simulink model "FSK"  (R2019a)
settings: Solver=VariableStepAuto  StartTime=0.0  StopTime=10.0  MaxStep=0.0001  RelTol=1e-3
libraries: dsparch4 x2, commchan3 x1, commrandsrc3 x1
settings Model: Creator=Lenovo  LastModifiedBy=MOSA

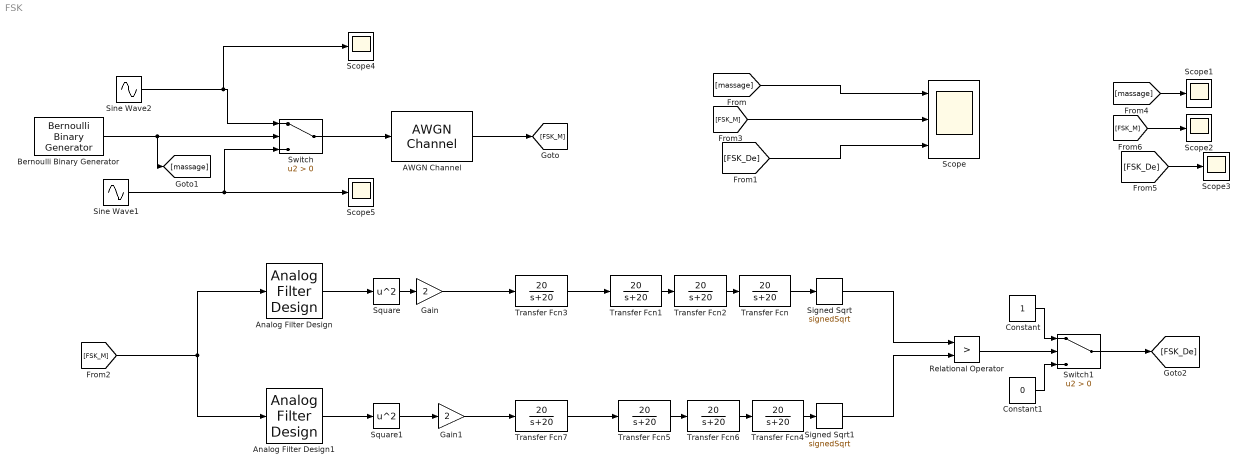
== system FSK ==
  AWGN Channel : commchan3/AWGN Channel  InputProcessing=Columns as channels (frame based)  seed=67  noiseMode="Signal to noise ratio  (SNR)"  EbNodB=10  EsNodB=10  SNRdB=10  bitsPerSym=1  Ps=1  Tsym=1  variance=1
  Analog Filter Design : dsparch4/Analog Filter Design  method=Butterworth  filttype=Bandpass  N=8  Wlo=50  Whi=200  Rp=2  Rs=40
  Analog Filter Design1 : dsparch4/Analog Filter Design  method=Butterworth  filttype=Bandpass  N=8  Wlo=2  Whi=50  Rp=2  Rs=40
  Bernoulli Binary Generator : commrandsrc3/Bernoulli Binary Generator  ProbabilityOfZero=0.5  SeedSource=Parameter  Seed=67  SampleTime=0.4  SamplesPerFrame=1  OutputDataType=double  SimulateUsing=Interpreted execution
  Constant : Constant
  Constant1 : Constant  Value=0
  Gain : Gain  Gain=2
  Gain1 : Gain  Gain=2
  Relational Operator : RelationalOperator  Operator=>  OutDataTypeStr=boolean  RndMeth=Simplest
  Scope : Scope  NumInputPorts=3
  Scope{1..5} (5 alike) : Scope
  Signed Sqrt : Sqrt  Operator=signedSqrt  SaturateOnIntegerOverflow=on
  Signed Sqrt1 : Sqrt  Operator=signedSqrt  SaturateOnIntegerOverflow=on
  Sine Wave1 : Sin  Frequency=31.4  SampleTime=0
  Sine Wave2 : Sin  Frequency=94.2  SampleTime=0
  Square : Math  Operator=square  SaturateOnIntegerOverflow=on
  Square1 : Math  Operator=square  SaturateOnIntegerOverflow=on
  Switch : Switch  Criteria=u2 > Threshold
  Switch1 : Switch  Criteria=u2 > Threshold
  Transfer Fcn{,1..7} (8 alike) : TransferFcn  Numerator=[20]  Denominator=[1 20]
  wires:
  Sine Wave2/1 -> Scope4/1, Switch/1
  Bernoulli Binary Generator/1 -> Switch/2, [massage]
  Sine Wave1/1 -> Switch/3, Scope5/1
  Square/1 -> Gain/1
  Transfer Fcn/1 -> Signed Sqrt/1
  Transfer Fcn1/1 -> Transfer Fcn2/1
  Transfer Fcn2/1 -> Transfer Fcn/1
  Gain/1 -> Transfer Fcn3/1
  Transfer Fcn6/1 -> Transfer Fcn4/1
  Transfer Fcn4/1 -> Signed Sqrt1/1
  Transfer Fcn5/1 -> Transfer Fcn6/1
  Square1/1 -> Gain1/1
  Gain1/1 -> Transfer Fcn7/1
  Analog Filter Design1/1 -> Square1/1
  Analog Filter Design/1 -> Square/1
  Constant/1 -> Switch1/1
  Constant1/1 -> Switch1/3
  Relational Operator/1 -> Switch1/2
  [FSK_M] -> Analog Filter Design/1, Analog Filter Design1/1
  Switch1/1 -> [FSK_De]
  Switch/1 -> AWGN Channel/1
  Transfer Fcn7/1 -> Transfer Fcn5/1
  Transfer Fcn3/1 -> Transfer Fcn1/1
  AWGN Channel/1 -> [FSK_M]
  Signed Sqrt/1 -> Relational Operator/1
  Signed Sqrt1/1 -> Relational Operator/2
  [massage] -> Scope/1
  [FSK_M] -> Scope/2
  [FSK_De] -> Scope/3
  [massage] -> Scope1/1
  [FSK_M] -> Scope2/1
  [FSK_De] -> Scope3/1
